simulink model "Torque_Vectoring_Schanzer20"  (R2018a)
settings: Solver=ode15s  StartTime=0.01  StopTime=inf  RelTol=1e-3  EnableMultiTasking=on
libraries: CarMaker4SL x8, dspstat3 x5, simulink x2
(part 2 of 3)

== system Torque_Vectoring_Schanzer20/CarMaker/IPG Vehicle/CarAndTrailer/Forces/Tires ==
  note: The TireXX_Out signals will only be used if FileIdent is "CarMaker-Tire-CM4SL" in the tire parameter file!
      | An example parameter file can be found in Data/Tire/DT_CM4SL_UserTire.
  Sync_In : Inport
  TireFL_In : Inport  Port=2
  TireFR_In : Inport  Port=3
  TireRL_In : Inport  Port=4
  TireRR_In : Inport  Port=5
  Bus Creator{1..4} (4 alike) : BusCreator  Inputs=11
  Demux{1..3,8} (4 alike) : Demux  Outputs=7
  TireFL : Subsystem
  TireFR : Subsystem
  TireRL : Subsystem
  TireRR : Subsystem
  TireFL_Out : Outport
  TireFR_Out : Outport  Port=2
  TireRL_Out : Outport  Port=3
  TireRR_Out : Outport  Port=4
  wires:
  Sync_In/1 -> TireRR/1(Sync_In), TireRL/1(Sync_In), TireFR/1(Sync_In), TireFL/1(Sync_In)
  Bus Creator4/1 -> TireRR_Out/1
  Bus Creator2/1 -> TireRL_Out/1
  Bus Creator1/1 -> TireFR_Out/1
  Demux3/5 -> TireRR/6(Rim_turnv)  "Tire_In Rim_turnv"
  Demux3/4 -> TireRR/5(Rim_rotv)  "Tire_In Rim_rotv"
  Demux3/1 -> TireRR/2(Load)  "Tire_In Load"
  Demux3/7 -> TireRR/8(muRoad)  "Tire_In mu"
  Demux3/6 -> TireRR/7(InclinAngle)  "Tire_In Camber"
  Demux3/2 -> TireRR/3(vxtrans)  "Tire_In vxtrans"
  Demux3/3 -> TireRR/4(vytrans)  "Tire_In vytrans"
  TireRR/11(AlignTrq) -> Bus Creator4/11  "Tire_Out AlignTrq"
  TireRR/10(RollResist) -> Bus Creator4/10  "Tire_Out RollResist"
  TireRR/9(OverturnTrq) -> Bus Creator4/9  "Tire_Out OverturnTrq"
  TireRR/8(LoadFrc) -> Bus Creator4/8  "Tire_Out LoadFrc"
  TireRR/7(SideFrc) -> Bus Creator4/7  "Tire_Out SideFrc"
  TireRR/6(LongFrc) -> Bus Creator4/6  "Tire_Out LongFrc"
  TireRR/5(vBelt) -> Bus Creator4/5  "Tire_Out vBelt"
  TireRR/4(rBelt_eff) -> Bus Creator4/4  "Tire_Out rBelt_eff"
  TireRR/3(TurnSlp) -> Bus Creator4/3  "Tire_Out TurnSlp"
  TireRR/1(Slp) -> Bus Creator4/1  "Tire_Out Slp"
  TireRR/2(Alpha) -> Bus Creator4/2  "Tire_Out Alpha"
  Demux2/5 -> TireRL/6(Rim_turnv)  "Tire_In Rim_turnv"
  Demux2/4 -> TireRL/5(Rim_rotv)  "Tire_In Rim_rotv"
  Demux2/1 -> TireRL/2(Load)  "Tire_In Load"
  Demux2/7 -> TireRL/8(muRoad)  "Tire_In mu"
  Demux2/6 -> TireRL/7(InclinAngle)  "Tire_In Camber"
  Demux2/2 -> TireRL/3(vxtrans)  "Tire_In vxtrans"
  Demux2/3 -> TireRL/4(vytrans)  "Tire_In vytrans"
  TireRL/11(AlignTrq) -> Bus Creator2/11  "Tire_Out AlignTrq"
  TireRL/10(RollResist) -> Bus Creator2/10  "Tire_Out RollResist"
  TireRL/9(OverturnTrq) -> Bus Creator2/9  "Tire_Out OverturnTrq"
  TireRL/8(LoadFrc) -> Bus Creator2/8  "Tire_Out LoadFrc"
  TireRL/7(SideFrc) -> Bus Creator2/7  "Tire_Out SideFrc"
  TireRL/6(LongFrc) -> Bus Creator2/6  "Tire_Out LongFrc"
  TireRL/5(vBelt) -> Bus Creator2/5  "Tire_Out vBelt"
  TireRL/4(rBelt_eff) -> Bus Creator2/4  "Tire_Out rBelt_eff"
  TireRL/3(TurnSlp) -> Bus Creator2/3  "Tire_Out TurnSlp"
  TireRL/1(Slp) -> Bus Creator2/1  "Tire_Out Slp"
  TireRL/2(Alpha) -> Bus Creator2/2  "Tire_Out Alpha"
  Demux1/5 -> TireFR/6(Rim_turnv)  "Tire_In Rim_turnv"
  Demux1/4 -> TireFR/5(Rim_rotv)  "Tire_In Rim_rotv"
  Demux1/1 -> TireFR/2(Load)  "Tire_In Load"
  Demux1/7 -> TireFR/8(muRoad)  "Tire_In mu"
  Demux1/6 -> TireFR/7(InclinAngle)  "Tire_In Camber"
  Demux1/2 -> TireFR/3(vxtrans)  "Tire_In vxtrans"
  Demux1/3 -> TireFR/4(vytrans)  "Tire_In vytrans"
  TireFR/11(AlignTrq) -> Bus Creator1/11  "Tire_Out AlignTrq"
  TireFR/10(RollResist) -> Bus Creator1/10  "Tire_Out RollResist"
  TireFR/9(OverturnTrq) -> Bus Creator1/9  "Tire_Out OverturnTrq"
  TireFR/8(LoadFrc) -> Bus Creator1/8  "Tire_Out LoadFrc"
  TireFR/7(SideFrc) -> Bus Creator1/7  "Tire_Out SideFrc"
  TireFR/6(LongFrc) -> Bus Creator1/6  "Tire_Out LongFrc"
  TireFR/5(vBelt) -> Bus Creator1/5  "Tire_Out vBelt"
  TireFR/4(rBelt_eff) -> Bus Creator1/4  "Tire_Out rBelt_eff"
  TireFR/3(TurnSlp) -> Bus Creator1/3  "Tire_Out TurnSlp"
  TireFR/1(Slp) -> Bus Creator1/1  "Tire_Out Slp"
  TireFR/2(Alpha) -> Bus Creator1/2  "Tire_Out Alpha"
  Demux8/5 -> TireFL/6(Rim_turnv)  "Tire_In Rim_turnv"
  Demux8/4 -> TireFL/5(Rim_rotv)  "Tire_In Rim_rotv"
  TireFL_In/1 -> Demux8/1
  Demux8/1 -> TireFL/2(Load)  "Tire_In Load"
  Demux8/7 -> TireFL/8(muRoad)  "Tire_In mu"
  Demux8/6 -> TireFL/7(InclinAngle)  "Tire_In Camber"
  Demux8/2 -> TireFL/3(vxtrans)  "Tire_In vxtrans"
  Demux8/3 -> TireFL/4(vytrans)  "Tire_In vytrans"
  TireFL/11(AlignTrq) -> Bus Creator3/11  "Tire_Out AlignTrq"
  TireFL/10(RollResist) -> Bus Creator3/10  "Tire_Out RollResist"
  TireFL/9(OverturnTrq) -> Bus Creator3/9  "Tire_Out OverturnTrq"
  TireFL/8(LoadFrc) -> Bus Creator3/8  "Tire_Out LoadFrc"
  TireFL/7(SideFrc) -> Bus Creator3/7  "Tire_Out SideFrc"
  TireFL/6(LongFrc) -> Bus Creator3/6  "Tire_Out LongFrc"
  TireFL/5(vBelt) -> Bus Creator3/5  "Tire_Out vBelt"
  TireFL/4(rBelt_eff) -> Bus Creator3/4  "Tire_Out rBelt_eff"
  TireFL/3(TurnSlp) -> Bus Creator3/3  "Tire_Out TurnSlp"
  TireFL/1(Slp) -> Bus Creator3/1  "Tire_Out Slp"
  TireFL/2(Alpha) -> Bus Creator3/2  "Tire_Out Alpha"
  Bus Creator3/1 -> TireFL_Out/1
  TireFR_In/1 -> Demux1/1
  TireRL_In/1 -> Demux2/1
  TireRR_In/1 -> Demux3/1

== system Torque_Vectoring_Schanzer20/CarMaker/IPG Vehicle/CarAndTrailer/Forces/Vehicle Forces ==
  Sync_In : Inport
  Bus Creator1 : BusCreator  Inputs=12
  Bus Creator8 : BusCreator  Inputs=16
  BusCreator1 : BusCreator  Inputs=4
  BusCreator2 : BusCreator  Inputs=9
  Demux : Demux  Outputs=16
  Demux1 : Demux  Outputs=12
  Demux2 : Demux  Outputs=13
  Forces : S-Function  FunctionName=CM_Sfun  Parameters='Forces'  SFunctionDeploymentMode=off  EnableBusSupport=off
  Terminator : Terminator
  Sync_Out : Outport
  Car.Virtual : Outport  Port=2
  Car.Aero : Outport  Port=3
  Car.Load : Outport  Port=4
  wires:
  BusCreator1/1 -> Terminator/1  "Aero IF (in)"
  Demux2/13 -> BusCreator2/9  "car Aero Trq_1 z"
  Demux2/12 -> BusCreator2/8  "car Aero Trq_1 y"
  Demux2/11 -> BusCreator2/7  "car Aero Trq_1 x"
  Demux2/10 -> BusCreator2/6  "car Aero Frc_1 z"
  Demux2/9 -> BusCreator2/5  "car Aero Frc_1 y"
  Demux2/8 -> BusCreator2/4  "car Aero Frc_1 x"
  Demux2/7 -> BusCreator2/3  "car Aero PoA_1 z"
  Demux2/6 -> BusCreator2/2  "car Aero PoA_1 y"
  Demux2/5 -> BusCreator2/1  "car Aero PoA_1 x"
  Demux2/4 -> BusCreator1/4  "car Aero tau_1"
  Demux2/3 -> BusCreator1/3  "car Aero ApproachVel_1 z"
  Demux2/2 -> BusCreator1/2  "car Aero ApproachVel_1 y"
  Demux2/1 -> BusCreator1/1  "car Aero ApproachVel_1 x"
  Demux/16 -> Bus Creator8/16  "Car Load_3 tz"
  Demux/15 -> Bus Creator8/15  "Car Load_3 ty"
  Demux/14 -> Bus Creator8/14  "Car Load_3 tx"
  Demux/13 -> Bus Creator8/13  "Car Load_3 mass"
  Demux1/12 -> Bus Creator1/12  "Car Virtual Trq_0 z"
  Demux1/11 -> Bus Creator1/11  "Car Virtual Trq_0 y"
  Demux1/10 -> Bus Creator1/10  "Car Virtual Trq_0 x"
  Demux1/9 -> Bus Creator1/9  "Car Virtual Trq_1 z"
  Demux1/8 -> Bus Creator1/8  "Car Virtual Trq_1 y"
  Demux1/7 -> Bus Creator1/7  "Car Virtual Trq_1 x"
  Demux1/6 -> Bus Creator1/6  "Car Virtual Frc_0 z"
  Demux1/5 -> Bus Creator1/5  "Car Virtual Frc_0 y"
  Demux1/4 -> Bus Creator1/4  "Car Virtual Frc_0 x"
  Sync_In/1 -> Forces/1
  Forces/1 -> Sync_Out/1
  BusCreator2/1 -> Car.Aero/1
  Demux1/1 -> Bus Creator1/1  "Car Virtual Frc_1 x"
  Demux1/2 -> Bus Creator1/2  "Car Virtual Frc_1 y"
  Demux1/3 -> Bus Creator1/3  "Car Virtual Frc_1 z"
  Forces/3 -> Demux2/1
  Forces/2 -> Demux1/1
  Bus Creator1/1 -> Car.Virtual/1
  Bus Creator8/1 -> Car.Load/1
  Demux/1 -> Bus Creator8/1  "Car Load_0 mass"
  Demux/2 -> Bus Creator8/2  "Car Load_0 tx"
  Demux/3 -> Bus Creator8/3  "Car Load_0 ty"
  Demux/4 -> Bus Creator8/4  "Car Load_0 tz"
  Demux/5 -> Bus Creator8/5  "Car Load_1 mass"
  Demux/6 -> Bus Creator8/6  "Car Load_1 tx"
  Demux/7 -> Bus Creator8/7  "Car Load_1 ty"
  Demux/8 -> Bus Creator8/8  "Car Load_1 tz"
  Demux/9 -> Bus Creator8/9  "Car Load_2 mass"
  Demux/10 -> Bus Creator8/10  "Car Load_2 tx"
  Demux/11 -> Bus Creator8/11  "Car Load_2 ty"
  Demux/12 -> Bus Creator8/12  "Car Load_2 tz"
  Forces/4 -> Demux/1

== system Torque_Vectoring_Schanzer20/CarMaker/IPG Vehicle/CarAndTrailer/Trailer/CreateBus Car.Hitch.FrcTrq ==
  In1 : Inport
  Bus Creator7 : BusCreator  Inputs=6
  Demux7 : Demux  Outputs=6
  Out1 : Outport
  wires:
  In1/1 -> Demux7/1
  Bus Creator7/1 -> Out1/1
  Demux7/6 -> Bus Creator7/6  "Car Hitch Trq2Car z"
  Demux7/5 -> Bus Creator7/5  "Car Hitch Trq2Car y"
  Demux7/4 -> Bus Creator7/4  "Car Hitch Trq2Car x"
  Demux7/3 -> Bus Creator7/3  "Car Hitch Frc2Car z"
  Demux7/2 -> Bus Creator7/2  "Car Hitch Frc2Car y"
  Demux7/1 -> Bus Creator7/1  "Car Hitch Frc2Car x"

== system Torque_Vectoring_Schanzer20/CarMaker/IPG Vehicle/CarAndTrailer/Trailer/CreateBus Vhcl.Motion ==
  In1 : Inport
  BusCreator : BusCreator  Inputs=15
  Demux : Demux  Outputs=15
  Scope : Scope
  Out1 : Outport
  Out2 : Outport  Port=2
  Out3 : Outport  Port=3
  wires:
  Demux/15 -> BusCreator/15  "Vhcl YawAcc"
  Demux/14 -> Scope/1, Out3/1, BusCreator/14  "Vhcl YawVel"
  Demux/13 -> BusCreator/13  "Vhcl Yaw"
  Demux/12 -> BusCreator/12  "Vhcl PitchAcc"
  Demux/11 -> BusCreator/11  "Vhcl PitchVel"
  Demux/10 -> BusCreator/10  "Vhcl Pitch"
  Demux/9 -> BusCreator/9  "Vhcl RollAcc"
  Demux/8 -> BusCreator/8  "Vhcl RollVel"
  Demux/7 -> BusCreator/7  "Vhcl Roll"
  Demux/6 -> BusCreator/6  "Vhcl Hitch_Pos z"
  Demux/5 -> BusCreator/5  "Vhcl Hitch_Pos y"
  Demux/4 -> BusCreator/4  "Vhcl Hitch_Pos x"
  Demux/3 -> BusCreator/3  "Vhcl sRoad"
  Demux/2 -> BusCreator/2  "Vhcl Distance"
  Demux/1 -> Out2/1, BusCreator/1  "Vhcl v"
  In1/1 -> Demux/1
  BusCreator/1 -> Out1/1

== system Torque_Vectoring_Schanzer20/CarMaker/IPG Vehicle/CarAndTrailer/Trailer/CreateBus Vhcl.PoI ==
  In1 : Inport
  Bus Creator3 : BusCreator  Inputs=18
  Demux3 : Demux  Outputs=18
  Out1 : Outport
  Out2 : Outport  Port=2
  wires:
  Demux3/18 -> Bus Creator3/18  "Vhcl PoI_GCS Elev"
  Demux3/17 -> Bus Creator3/17  "Vhcl PoI_GCS Lat"
  Demux3/16 -> Bus Creator3/16  "Vhcl PoI_GCS Long"
  Demux3/15 -> Bus Creator3/15  "Vhcl PoI_Acc_1 z"
  Demux3/14 -> Bus Creator3/14  "Vhcl PoI_Acc_1 y"
  Demux3/13 -> Out2/1, Bus Creator3/13  "Vhcl PoI_Acc_1 x"
  Demux3/12 -> Bus Creator3/12  "Vhcl PoI_Vel_1 z"
  Demux3/11 -> Bus Creator3/11  "Vhcl PoI_Vel_1 y"
  Demux3/10 -> Bus Creator3/10  "Vhcl PoI_Vel_1 x"
  Demux3/9 -> Bus Creator3/9  "Vhcl PoI_Acc z"
  Demux3/8 -> Bus Creator3/8  "Vhcl PoI_Acc y"
  Demux3/7 -> Bus Creator3/7  "Vhcl PoI_Acc x"
  Demux3/6 -> Bus Creator3/6  "Vhcl PoI_Vel z"
  Demux3/5 -> Bus Creator3/5  "Vhcl PoI_Vel y"
  Demux3/4 -> Bus Creator3/4  "Vhcl PoI_Vel x"
  Demux3/3 -> Bus Creator3/3  "Vhcl PoI_Pos z"
  Demux3/2 -> Bus Creator3/2  "Vhcl PoI_Pos y"
  In1/1 -> Demux3/1
  Bus Creator3/1 -> Out1/1
  Demux3/1 -> Bus Creator3/1  "Vhcl PoI_Pos x"

== system Torque_Vectoring_Schanzer20/CarMaker/IPG Vehicle/CarAndTrailer/Trailer/CreateBus Vhcl.Steering ==
  In1 : Inport
  Bus Creator3 : BusCreator  Inputs=4
  Demux : Demux
  Out1 : Outport
  Out2 : Outport  Port=2
  wires:
  Bus Creator3/1 -> Out1/1
  Demux/1 -> Out2/1, Bus Creator3/1  "Vehicle Steering Ang"
  Demux/3 -> Bus Creator3/3  "Vhcl Steering AngAcc"
  Demux/2 -> Bus Creator3/2  "Vhcl Steering AngVel"
  Demux/4 -> Bus Creator3/4  "Vhcl Steering Trq"
  In1/1 -> Demux/1

== system Torque_Vectoring_Schanzer20/CarMaker/IPG Vehicle/CarAndTrailer/Trailer/CreateBus Vhcl.Wheel.FL ==
  In1 : Inport
  Bus Creator3 : BusCreator  Inputs=14
  Demux3 : Demux  Outputs=14
  Out1 : Outport
  wires:
  Demux3/14 -> Bus Creator3/14  "Vhcl Wheel FL Trq_WhlBearing"
  Demux3/12 -> Bus Creator3/12  "Vhcl Wheel FL SideSlip"
  Demux3/11 -> Bus Creator3/11  "Vhcl Wheel FL LongSlip"
  Demux3/10 -> Bus Creator3/10  "Vhcl Wheel FL vBelt"
  Demux3/9 -> Bus Creator3/9  "Vhcl Wheel FL Fz"
  Demux3/8 -> Bus Creator3/8  "Vhcl Wheel FL Fy"
  Demux3/7 -> Bus Creator3/7  "Vhcl Wheel FL Fx"
  Demux3/6 -> Bus Creator3/6  "Vhcl Wheel FL r_zxy z"
  Demux3/5 -> Bus Creator3/5  "Vhcl Wheel FL r_zxy y"
  Demux3/4 -> Bus Creator3/4  "Vhcl Wheel FL r_zxy x"
  Demux3/3 -> Bus Creator3/3  "Vhcl Wheel FL t z"
  Demux3/2 -> Bus Creator3/2  "Vhcl Wheel FL t y"
  In1/1 -> Demux3/1
  Bus Creator3/1 -> Out1/1
  Demux3/1 -> Bus Creator3/1  "Vhcl Wheel FL t x"
  Demux3/13 -> Bus Creator3/13  "Vhcl Wheel FL Trq_T2W"

== system Torque_Vectoring_Schanzer20/CarMaker/IPG Vehicle/CarAndTrailer/Trailer/CreateBus Vhcl.Wheel.FR ==
  In1 : Inport
  Bus Creator3 : BusCreator  Inputs=14
  Demux3 : Demux  Outputs=14
  Out1 : Outport
  wires:
  Demux3/14 -> Bus Creator3/14  "Vhcl Wheel FR Trq_WhlBearing"
  Demux3/12 -> Bus Creator3/12  "Vhcl Wheel FR SideSlip"
  Demux3/11 -> Bus Creator3/11  "Vhcl Wheel FR LongSlip"
  Demux3/10 -> Bus Creator3/10  "Vhcl Wheel FR vBelt"
  Demux3/9 -> Bus Creator3/9  "Vhcl Wheel FR Fz"
  Demux3/8 -> Bus Creator3/8  "Vhcl Wheel FR Fy"
  Demux3/7 -> Bus Creator3/7  "Vhcl Wheel FR Fx"
  Demux3/6 -> Bus Creator3/6  "Vhcl Wheel FR r_zxy z"
  Demux3/5 -> Bus Creator3/5  "Vhcl Wheel FR r_zxy y"
  Demux3/4 -> Bus Creator3/4  "Vhcl Wheel FR r_zxy x"
  Demux3/3 -> Bus Creator3/3  "Vhcl Wheel FR t z"
  Demux3/2 -> Bus Creator3/2  "Vhcl Wheel FR t y"
  In1/1 -> Demux3/1
  Bus Creator3/1 -> Out1/1
  Demux3/1 -> Bus Creator3/1  "Vhcl Wheel FR t x"
  Demux3/13 -> Bus Creator3/13  "Vhcl Wheel FR Trq_T2W"

== system Torque_Vectoring_Schanzer20/CarMaker/IPG Vehicle/CarAndTrailer/Trailer/CreateBus Vhcl.Wheel.RL ==
  In1 : Inport
  Bus Creator3 : BusCreator  Inputs=14
  Demux3 : Demux  Outputs=14
  Out1 : Outport
  wires:
  Demux3/14 -> Bus Creator3/14  "Vhcl Wheel RL Trq_WhlBearing"
  Demux3/12 -> Bus Creator3/12  "Vhcl Wheel RL SideSlip"
  Demux3/11 -> Bus Creator3/11  "Vhcl Wheel RL LongSlip"
  Demux3/10 -> Bus Creator3/10  "Vhcl Wheel RL vBelt"
  Demux3/9 -> Bus Creator3/9  "Vhcl Wheel RL Fz"
  Demux3/8 -> Bus Creator3/8  "Vhcl Wheel RL Fy"
  Demux3/7 -> Bus Creator3/7  "Vhcl Wheel RL Fx"
  Demux3/6 -> Bus Creator3/6  "Vhcl Wheel RL r_zxy z"
  Demux3/5 -> Bus Creator3/5  "Vhcl Wheel RL r_zxy y"
  Demux3/4 -> Bus Creator3/4  "Vhcl Wheel RL r_zxy x"
  Demux3/3 -> Bus Creator3/3  "Vhcl Wheel RL t z"
  Demux3/2 -> Bus Creator3/2  "Vhcl Wheel RL t y"
  In1/1 -> Demux3/1
  Bus Creator3/1 -> Out1/1
  Demux3/1 -> Bus Creator3/1  "Vhcl Wheel RL t x"
  Demux3/13 -> Bus Creator3/13  "Vhcl Wheel RL Trq_T2W"

== system Torque_Vectoring_Schanzer20/CarMaker/IPG Vehicle/CarAndTrailer/Trailer/CreateBus Vhcl.Wheel.RR ==
  In1 : Inport
  Bus Creator3 : BusCreator  Inputs=14
  Demux3 : Demux  Outputs=14
  Out1 : Outport
  wires:
  Demux3/14 -> Bus Creator3/14  "Vhcl Wheel RR Trq_WhlBearing"
  Demux3/12 -> Bus Creator3/12  "Vhcl Wheel RR SideSlip"
  Demux3/11 -> Bus Creator3/11  "Vhcl Wheel RR LongSlip"
  Demux3/10 -> Bus Creator3/10  "Vhcl Wheel RR vBelt"
  Demux3/9 -> Bus Creator3/9  "Vhcl Wheel RR Fz"
  Demux3/8 -> Bus Creator3/8  "Vhcl Wheel RR Fy"
  Demux3/7 -> Bus Creator3/7  "Vhcl Wheel RR Fx"
  Demux3/6 -> Bus Creator3/6  "Vhcl Wheel RR r_zxy z"
  Demux3/5 -> Bus Creator3/5  "Vhcl Wheel RR r_zxy y"
  Demux3/4 -> Bus Creator3/4  "Vhcl Wheel RR r_zxy x"
  Demux3/3 -> Bus Creator3/3  "Vhcl Wheel RR t z"
  Demux3/2 -> Bus Creator3/2  "Vhcl Wheel RR t y"
  In1/1 -> Demux3/1
  Bus Creator3/1 -> Out1/1
  Demux3/1 -> Bus Creator3/1  "Vhcl Wheel RR t x"
  Demux3/13 -> Bus Creator3/13  "Vhcl Wheel RR Trq_T2W"

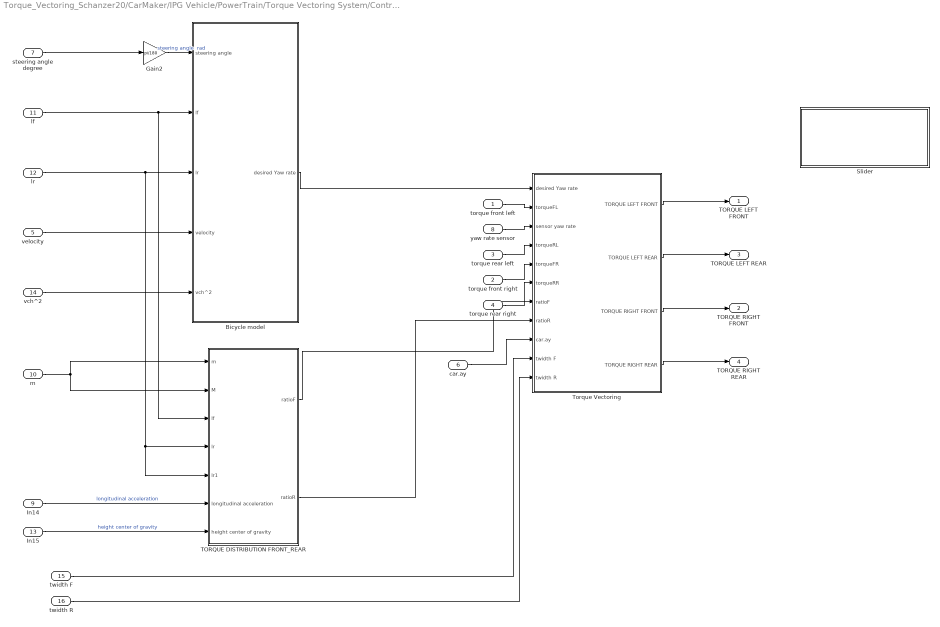
== system Torque_Vectoring_Schanzer20/CarMaker/IPG Vehicle/PowerTrain/Torque Vectoring System/Controller Logic1 ==
  torque front left : Inport
  torque front right : Inport  Port=2
  torque rear left : Inport  Port=3
  torque rear right : Inport  Port=4
  velocity : Inport  Port=5
  car.ay : Inport  Port=6
  steering angle degree : Inport  Port=7
  yaw rate sensor : Inport  Port=8
  In14 : Inport  Port=9
  m : Inport  Port=10
  lf : Inport  Port=11
  lr : Inport  Port=12
  In15 : Inport  Port=13
  vch^2 : Inport  Port=14
  twidth F : Inport  Port=15
  twidth R : Inport  Port=16
  Bicycle model : Subsystem
  Gain2 : Gain  Gain=pi/180
  Slider : Subsystem  DialogController=hmiCreateDDGDialog  IsWebBlock=on  mask(MWDashboardBlock){webBlockId=59816ab4-1199-4927-a44c-d672ac8afe40, webBlockType=slider, ShowInLibBrowser=on, ShowInitialText=on, HMISrcModelName=Torque_Vectoring_Schanzer20}
      mask prompts: webBlockId "WebBlock Id"; webBlockType "WebBlock Type"; HMISrcModelName "Source Model"
      mask help: SimulinkHMI:dialogs:SliderDialogDesc
      mask Help: helpview([docroot '/mapfiles/simulink.map'], 'hmi_slider')
      mask Display:
      | if strcmp(get_param(bdroot(gcb),'BlockDiagramType'), 'library')
      |     image([(matlabroot) '/toolbox/simulink/hmi/icons/Slider.png']);
      | end
  TORQUE DISTRIBUTION FRONT_REAR : Subsystem
  Torque Vectoring : Subsystem
  TORQUE LEFT FRONT : Outport
  TORQUE RIGHT FRONT : Outport  Port=2
  TORQUE LEFT REAR : Outport  Port=3
  TORQUE RIGHT REAR : Outport  Port=4
  wires:
  Gain2/1 -> Bicycle model/1(steering angle)  "steering angle  rad"
  steering angle degree/1 -> Gain2/1
  lf/1 -> TORQUE DISTRIBUTION FRONT_REAR/3(lf), Bicycle model/2(lf)
  m/1 -> TORQUE DISTRIBUTION FRONT_REAR/2(M), TORQUE DISTRIBUTION FRONT_REAR/1(m)
  lr/1 -> TORQUE DISTRIBUTION FRONT_REAR/5(lr1), TORQUE DISTRIBUTION FRONT_REAR/4(lr), Bicycle model/3(lr)
  In14/1 -> TORQUE DISTRIBUTION FRONT_REAR/6(longitudinal acceleration)  "longitudinal acceleration"
  In15/1 -> TORQUE DISTRIBUTION FRONT_REAR/7(height center of gravity)  "height center of gravity"
  velocity/1 -> Bicycle model/4(velocity)
  Bicycle model/1(" desired Yaw rate") -> Torque Vectoring/1(desired Yaw rate)
  torque front left/1 -> Torque Vectoring/2(torqueFL)
  yaw rate sensor/1 -> Torque Vectoring/3(sensor yaw rate)
  torque rear left/1 -> Torque Vectoring/4(torqueRL)
  torque front right/1 -> Torque Vectoring/5(torqueFR)
  torque rear right/1 -> Torque Vectoring/6(torqueRR)
  TORQUE DISTRIBUTION FRONT_REAR/1(ratioF) -> Torque Vectoring/7(ratioF)
  TORQUE DISTRIBUTION FRONT_REAR/2(ratioR) -> Torque Vectoring/8(ratioR)
  Torque Vectoring/1(TORQUE LEFT FRONT) -> TORQUE LEFT FRONT/1
  Torque Vectoring/2(TORQUE LEFT REAR) -> TORQUE LEFT REAR/1
  Torque Vectoring/3(TORQUE RIGHT FRONT) -> TORQUE RIGHT FRONT/1
  Torque Vectoring/4(TORQUE RIGHT REAR) -> TORQUE RIGHT REAR/1
  car.ay/1 -> Torque Vectoring/9(car.ay)
  vch^2/1 -> Bicycle model/5(vch^2)
  twidth F/1 -> Torque Vectoring/10(twidth F)
  twidth R/1 -> Torque Vectoring/11(twidth R)

== system Torque_Vectoring_Schanzer20/CarMaker/IPG Vehicle/PowerTrain/Torque Vectoring System/activate system dependent1 ==
  In1 : Inport
  Constant1 : Constant  Value=0
  If : If  IfExpression=u1 > 0.1
  If Action Subsystem : Subsystem  TreatAsAtomicUnit=on
  If Action Subsystem1 : Subsystem  TreatAsAtomicUnit=on
  If Action Subsystem2 : Subsystem  TreatAsAtomicUnit=on
  If Action Subsystem3 : Subsystem  TreatAsAtomicUnit=on
  If1 : If  IfExpression=u1 < 1000
  Merge : Merge  InitialOutput=0
  Merge1 : Merge  InitialOutput=0
  Out1 : Outport
  wires:
  If Action Subsystem3/1(Out1) -> Merge1/2
  If/1 -> If Action Subsystem/Action
  Constant1/1 -> If Action Subsystem3/1(In1), If Action Subsystem1/1(In1)
  If Action Subsystem/1(Out1) -> Merge/1
  In1/1 -> If Action Subsystem/1(In1), If/1, If1/1
  If1/1 -> If Action Subsystem2/Action
  If Action Subsystem1/1(Out1) -> Merge/2
  If1/2 -> If Action Subsystem3/Action
  If/2 -> If Action Subsystem1/Action
  If Action Subsystem2/1(Out1) -> Merge1/1
  Merge/1 -> If Action Subsystem2/1(In1)
  Merge1/1 -> Out1/1

== system Torque_Vectoring_Schanzer20/CarMaker/IPG Vehicle/PowerTrain/Torque Vectoring System/activate system dependent2 ==
  In1 : Inport
  Constant1 : Constant  Value=0
  If : If  IfExpression=u1 > 0.1
  If Action Subsystem : Subsystem  TreatAsAtomicUnit=on
  If Action Subsystem1 : Subsystem  TreatAsAtomicUnit=on
  If Action Subsystem2 : Subsystem  TreatAsAtomicUnit=on
  If Action Subsystem3 : Subsystem  TreatAsAtomicUnit=on
  If1 : If  IfExpression=u1 < 1000
  Merge : Merge  InitialOutput=0
  Merge1 : Merge  InitialOutput=0
  Out1 : Outport
  wires:
  If Action Subsystem3/1(Out1) -> Merge1/2
  If/1 -> If Action Subsystem/Action
  Constant1/1 -> If Action Subsystem3/1(In1), If Action Subsystem1/1(In1)
  If Action Subsystem/1(Out1) -> Merge/1
  In1/1 -> If Action Subsystem/1(In1), If/1, If1/1
  If1/1 -> If Action Subsystem2/Action
  If Action Subsystem1/1(Out1) -> Merge/2
  If1/2 -> If Action Subsystem3/Action
  If/2 -> If Action Subsystem1/Action
  If Action Subsystem2/1(Out1) -> Merge1/1
  Merge/1 -> If Action Subsystem2/1(In1)
  Merge1/1 -> Out1/1

== system Torque_Vectoring_Schanzer20/CarMaker/IPG Vehicle/PowerTrain/Torque Vectoring System/activate system dependent3 ==
  In1 : Inport
  Constant1 : Constant  Value=0
  If : If  IfExpression=u1 > 0.1
  If Action Subsystem : Subsystem  TreatAsAtomicUnit=on
  If Action Subsystem1 : Subsystem  TreatAsAtomicUnit=on
  If Action Subsystem2 : Subsystem  TreatAsAtomicUnit=on
  If Action Subsystem3 : Subsystem  TreatAsAtomicUnit=on
  If1 : If  IfExpression=u1 < 1000
  Merge : Merge  InitialOutput=0
  Merge1 : Merge  InitialOutput=0
  Out1 : Outport
  wires:
  If Action Subsystem3/1(Out1) -> Merge1/2
  If/1 -> If Action Subsystem/Action
  Constant1/1 -> If Action Subsystem3/1(In1), If Action Subsystem1/1(In1)
  If Action Subsystem/1(Out1) -> Merge/1
  In1/1 -> If Action Subsystem/1(In1), If/1, If1/1
  If1/1 -> If Action Subsystem2/Action
  If Action Subsystem1/1(Out1) -> Merge/2
  If1/2 -> If Action Subsystem3/Action
  If/2 -> If Action Subsystem1/Action
  If Action Subsystem2/1(Out1) -> Merge1/1
  Merge/1 -> If Action Subsystem2/1(In1)
  Merge1/1 -> Out1/1

== system Torque_Vectoring_Schanzer20/CarMaker/IPG Vehicle/PowerTrain/Torque Vectoring System/activate system dependent5 ==
  In1 : Inport
  Constant1 : Constant
  If : If  IfExpression=u1 > 0.01
  If Action Subsystem : Subsystem  TreatAsAtomicUnit=on
  If Action Subsystem1 : Subsystem  TreatAsAtomicUnit=on
  If Action Subsystem2 : Subsystem  TreatAsAtomicUnit=on
  If Action Subsystem3 : Subsystem  TreatAsAtomicUnit=on
  If1 : If  IfExpression=u1 < 1000
  Merge : Merge  InitialOutput=0
  Merge1 : Merge  InitialOutput=0
  Out1 : Outport
  wires:
  If Action Subsystem3/1(Out1) -> Merge1/2
  If/1 -> If Action Subsystem/Action
  Constant1/1 -> If Action Subsystem3/1(In1), If Action Subsystem1/1(In1)
  If Action Subsystem/1(Out1) -> Merge/1
  In1/1 -> If Action Subsystem/1(In1), If/1, If1/1
  If1/1 -> If Action Subsystem2/Action
  If Action Subsystem1/1(Out1) -> Merge/2
  If1/2 -> If Action Subsystem3/Action
  If/2 -> If Action Subsystem1/Action
  If Action Subsystem2/1(Out1) -> Merge1/1
  Merge/1 -> If Action Subsystem2/1(In1)
  Merge1/1 -> Out1/1

== system Torque_Vectoring_Schanzer20/CarMaker/IPG Vehicle/PowerTrain/Torque Vectoring System/activate system dependent6 ==
  In1 : Inport
  Constant1 : Constant  Value=0
  If : If  IfExpression=u1 > 0.1
  If Action Subsystem : Subsystem  TreatAsAtomicUnit=on
  If Action Subsystem1 : Subsystem  TreatAsAtomicUnit=on
  If Action Subsystem2 : Subsystem  TreatAsAtomicUnit=on
  If Action Subsystem3 : Subsystem  TreatAsAtomicUnit=on
  If1 : If  IfExpression=u1 < 1000
  Merge : Merge  InitialOutput=0
  Merge1 : Merge  InitialOutput=0
  Out1 : Outport
  wires:
  If Action Subsystem3/1(Out1) -> Merge1/2
  If/1 -> If Action Subsystem/Action
  Constant1/1 -> If Action Subsystem3/1(In1), If Action Subsystem1/1(In1)
  If Action Subsystem/1(Out1) -> Merge/1
  In1/1 -> If Action Subsystem/1(In1), If/1, If1/1
  If1/1 -> If Action Subsystem2/Action
  If Action Subsystem1/1(Out1) -> Merge/2
  If1/2 -> If Action Subsystem3/Action
  If/2 -> If Action Subsystem1/Action
  If Action Subsystem2/1(Out1) -> Merge1/1
  Merge/1 -> If Action Subsystem2/1(In1)
  Merge1/1 -> Out1/1

== system Torque_Vectoring_Schanzer20/CarMaker/IPG Vehicle/PowerTrain/Torque Vectoring System/velocity estimation ==
  note: Assuming that angle of attack change rate is 0 -> steady state cornering (improvement would be including estimation of angle of attack (and change rate)
      | Checking of straight line noise of yaw rate sensor necessary to define a reasonable treshhold
  note: Ignore sensor offset; only switching when threshold is exceeded
  yaw rate : Inport
  centrifugal acceleration : Inport  Port=2
  Abs : Abs
  Abs1 : Abs
  Add : Sum
  Constant : Constant  Value=-1
  Constant1 : Constant  Value=-1
  Memory : Memory
  Sampling continous signal 50Hz1 : RateTransition  OutPortSampleTime=1/50
  Sampling continous signal 50Hz4 : RateTransition  OutPortSampleTime=1/50
  Switch1 : Switch  Criteria=u2 > Threshold  Threshold=0.05
  Switch2 : Switch  Criteria=u2 > Threshold  Threshold=0.1
  Switch3 : Switch
  v_viaYawRate_CentrifugalAcceleration : Subsystem
  Out1 : Outport
  wires:
  Add/1 -> Switch3/2
  Sampling continous signal 50Hz1/1 -> Switch1/2, Switch1/1
  Switch3/1 -> Out1/1, Memory/1  "velocity"
  Abs1/1 -> Sampling continous signal 50Hz4/1
  Switch1/1 -> Add/1, v_viaYawRate_CentrifugalAcceleration/1(YawRate)
  Sampling continous signal 50Hz4/1 -> Switch2/2, Switch2/1
  Memory/1 -> Switch3/3
  Abs/1 -> Sampling continous signal 50Hz1/1
  Constant1/1 -> Switch1/3
  yaw rate/1 -> Abs/1  "YawRate"
  v_viaYawRate_CentrifugalAcceleration/1(Out1) -> Switch3/1
  Constant/1 -> Switch2/3
  Switch2/1 -> Add/2, v_viaYawRate_CentrifugalAcceleration/2(ay)
  centrifugal acceleration/1 -> Abs1/1  "ay"

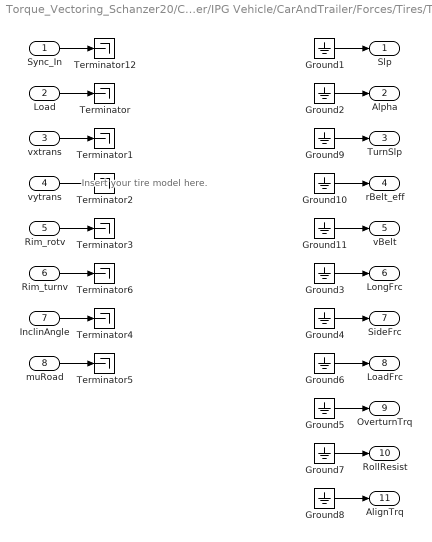
== system Torque_Vectoring_Schanzer20/CarMaker/IPG Vehicle/CarAndTrailer/Forces/Tires/TireFL ==
  note: Insert your tire model here.
  Sync_In : Inport
  Load : Inport  Port=2
  vxtrans : Inport  Port=3
  vytrans : Inport  Port=4
  Rim_rotv : Inport  Port=5
  Rim_turnv : Inport  Port=6
  InclinAngle : Inport  Port=7
  muRoad : Inport  Port=8
  Ground{1..11} (11 alike) : Ground
  Terminator{,1..6,12} (8 alike) : Terminator
  Slp : Outport
  Alpha : Outport  Port=2
  TurnSlp : Outport  Port=3
  rBelt_eff : Outport  Port=4
  vBelt : Outport  Port=5
  LongFrc : Outport  Port=6
  SideFrc : Outport  Port=7
  LoadFrc : Outport  Port=8
  OverturnTrq : Outport  Port=9
  RollResist : Outport  Port=10
  AlignTrq : Outport  Port=11
  wires:
  Ground11/1 -> vBelt/1
  Ground10/1 -> rBelt_eff/1
  Ground9/1 -> TurnSlp/1
  Rim_turnv/1 -> Terminator6/1
  Sync_In/1 -> Terminator12/1
  Ground2/1 -> Alpha/1
  Ground3/1 -> LongFrc/1
  Ground4/1 -> SideFrc/1
  Ground5/1 -> OverturnTrq/1
  vxtrans/1 -> Terminator1/1
  vytrans/1 -> Terminator2/1
  Rim_rotv/1 -> Terminator3/1
  InclinAngle/1 -> Terminator4/1
  muRoad/1 -> Terminator5/1
  Load/1 -> Terminator/1
  Ground1/1 -> Slp/1
  Ground6/1 -> LoadFrc/1
  Ground7/1 -> RollResist/1
  Ground8/1 -> AlignTrq/1

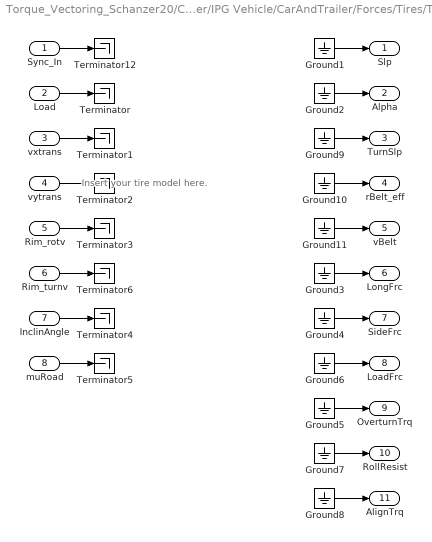
== system Torque_Vectoring_Schanzer20/CarMaker/IPG Vehicle/CarAndTrailer/Forces/Tires/TireFR ==
  note: Insert your tire model here.
  Sync_In : Inport
  Load : Inport  Port=2
  vxtrans : Inport  Port=3
  vytrans : Inport  Port=4
  Rim_rotv : Inport  Port=5
  Rim_turnv : Inport  Port=6
  InclinAngle : Inport  Port=7
  muRoad : Inport  Port=8
  Ground{1..11} (11 alike) : Ground
  Terminator{,1..6,12} (8 alike) : Terminator
  Slp : Outport
  Alpha : Outport  Port=2
  TurnSlp : Outport  Port=3
  rBelt_eff : Outport  Port=4
  vBelt : Outport  Port=5
  LongFrc : Outport  Port=6
  SideFrc : Outport  Port=7
  LoadFrc : Outport  Port=8
  OverturnTrq : Outport  Port=9
  RollResist : Outport  Port=10
  AlignTrq : Outport  Port=11
  wires:
  Ground11/1 -> vBelt/1
  Ground10/1 -> rBelt_eff/1
  Ground9/1 -> TurnSlp/1
  Rim_turnv/1 -> Terminator6/1
  Sync_In/1 -> Terminator12/1
  Ground2/1 -> Alpha/1
  Ground3/1 -> LongFrc/1
  Ground4/1 -> SideFrc/1
  Ground5/1 -> OverturnTrq/1
  vxtrans/1 -> Terminator1/1
  vytrans/1 -> Terminator2/1
  Rim_rotv/1 -> Terminator3/1
  InclinAngle/1 -> Terminator4/1
  muRoad/1 -> Terminator5/1
  Load/1 -> Terminator/1
  Ground1/1 -> Slp/1
  Ground6/1 -> LoadFrc/1
  Ground7/1 -> RollResist/1
  Ground8/1 -> AlignTrq/1

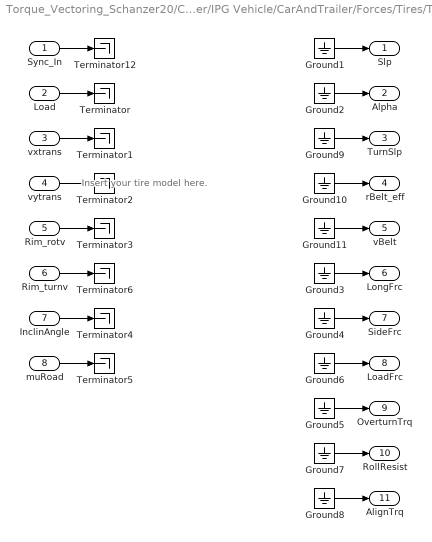
== system Torque_Vectoring_Schanzer20/CarMaker/IPG Vehicle/CarAndTrailer/Forces/Tires/TireRL ==
  note: Insert your tire model here.
  Sync_In : Inport
  Load : Inport  Port=2
  vxtrans : Inport  Port=3
  vytrans : Inport  Port=4
  Rim_rotv : Inport  Port=5
  Rim_turnv : Inport  Port=6
  InclinAngle : Inport  Port=7
  muRoad : Inport  Port=8
  Ground{1..11} (11 alike) : Ground
  Terminator{,1..6,12} (8 alike) : Terminator
  Slp : Outport
  Alpha : Outport  Port=2
  TurnSlp : Outport  Port=3
  rBelt_eff : Outport  Port=4
  vBelt : Outport  Port=5
  LongFrc : Outport  Port=6
  SideFrc : Outport  Port=7
  LoadFrc : Outport  Port=8
  OverturnTrq : Outport  Port=9
  RollResist : Outport  Port=10
  AlignTrq : Outport  Port=11
  wires:
  Ground11/1 -> vBelt/1
  Ground10/1 -> rBelt_eff/1
  Ground9/1 -> TurnSlp/1
  Rim_turnv/1 -> Terminator6/1
  Sync_In/1 -> Terminator12/1
  Ground2/1 -> Alpha/1
  Ground3/1 -> LongFrc/1
  Ground4/1 -> SideFrc/1
  Ground5/1 -> OverturnTrq/1
  vxtrans/1 -> Terminator1/1
  vytrans/1 -> Terminator2/1
  Rim_rotv/1 -> Terminator3/1
  InclinAngle/1 -> Terminator4/1
  muRoad/1 -> Terminator5/1
  Load/1 -> Terminator/1
  Ground1/1 -> Slp/1
  Ground6/1 -> LoadFrc/1
  Ground7/1 -> RollResist/1
  Ground8/1 -> AlignTrq/1

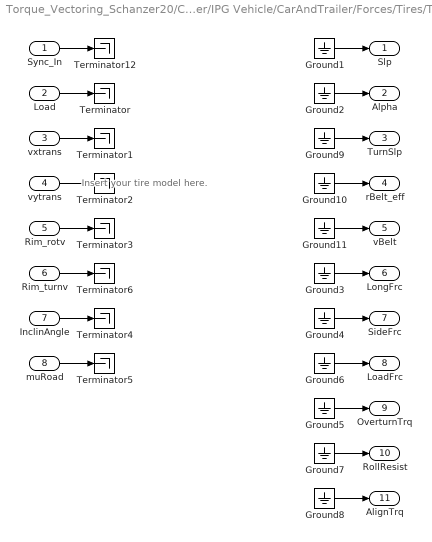
== system Torque_Vectoring_Schanzer20/CarMaker/IPG Vehicle/CarAndTrailer/Forces/Tires/TireRR ==
  note: Insert your tire model here.
  Sync_In : Inport
  Load : Inport  Port=2
  vxtrans : Inport  Port=3
  vytrans : Inport  Port=4
  Rim_rotv : Inport  Port=5
  Rim_turnv : Inport  Port=6
  InclinAngle : Inport  Port=7
  muRoad : Inport  Port=8
  Ground{1..11} (11 alike) : Ground
  Terminator{,1..6,12} (8 alike) : Terminator
  Slp : Outport
  Alpha : Outport  Port=2
  TurnSlp : Outport  Port=3
  rBelt_eff : Outport  Port=4
  vBelt : Outport  Port=5
  LongFrc : Outport  Port=6
  SideFrc : Outport  Port=7
  LoadFrc : Outport  Port=8
  OverturnTrq : Outport  Port=9
  RollResist : Outport  Port=10
  AlignTrq : Outport  Port=11
  wires:
  Ground11/1 -> vBelt/1
  Ground10/1 -> rBelt_eff/1
  Ground9/1 -> TurnSlp/1
  Rim_turnv/1 -> Terminator6/1
  Sync_In/1 -> Terminator12/1
  Ground2/1 -> Alpha/1
  Ground3/1 -> LongFrc/1
  Ground4/1 -> SideFrc/1
  Ground5/1 -> OverturnTrq/1
  vxtrans/1 -> Terminator1/1
  vytrans/1 -> Terminator2/1
  Rim_rotv/1 -> Terminator3/1
  InclinAngle/1 -> Terminator4/1
  muRoad/1 -> Terminator5/1
  Load/1 -> Terminator/1
  Ground1/1 -> Slp/1
  Ground6/1 -> LoadFrc/1
  Ground7/1 -> RollResist/1
  Ground8/1 -> AlignTrq/1

== system Torque_Vectoring_Schanzer20/CarMaker/IPG Vehicle/PowerTrain/Torque Vectoring System/Controller Logic1/Bicycle model ==
  steering angle : Inport
  lf : Inport  Port=2
  lr : Inport  Port=3
  velocity : Inport  Port=4
  vch^2 : Inport  Port=5
  Time delay : TransferFcn  Denominator=[0.08 1]
  linear bicycle model : Subsystem
  " desired Yaw rate" : Outport
  wires:
  lf/1 -> linear bicycle model/2(lf)
  steering angle/1 -> linear bicycle model/1(steering angle)
  lr/1 -> linear bicycle model/3(lr)
  velocity/1 -> linear bicycle model/4(velocity)
  Time delay/1 -> " desired Yaw rate"/1
  linear bicycle model/1(Yaw rate) -> Time delay/1
  vch^2/1 -> linear bicycle model/5(vch^2)

== system Torque_Vectoring_Schanzer20/CarMaker/IPG Vehicle/PowerTrain/Torque Vectoring System/Controller Logic1/Slider ==

== system Torque_Vectoring_Schanzer20/CarMaker/IPG Vehicle/PowerTrain/Torque Vectoring System/Controller Logic1/TORQUE DISTRIBUTION FRONT_REAR ==
  m : Inport
  M : Inport  Port=2
  lf : Inport  Port=3
  lr : Inport  Port=4
  lr1 : Inport  Port=5
  longitudinal acceleration : Inport  Port=6
  height center of gravity : Inport  Port=7
  Constant2 : Constant
  FRONTLOAD X : Subsystem
  LOADRATIO FRONT : Product  Inputs=*/
  LOADRATIO REAR : Sum  Inputs=+-
  REARLOAD x : Subsystem
  TOTAL WHEELLOAD : Sum
  ratioF : Outport
  ratioR : Outport  Port=2
  wires:
  REARLOAD x/1(L) -> FRONTLOAD X/5(L)
  TOTAL WHEELLOAD/1 -> LOADRATIO FRONT/2
  lf/1 -> REARLOAD x/2(lf)
  height center of gravity/1 -> REARLOAD x/5(height center of gravity), FRONTLOAD X/4(height center of gravity)
  m/1 -> FRONTLOAD X/1(m)
  FRONTLOAD X/1(normalloadF) -> TOTAL WHEELLOAD/1, LOADRATIO FRONT/1
  lr1/1 -> FRONTLOAD X/2(lr)
  M/1 -> REARLOAD x/1(M)
  lr/1 -> REARLOAD x/3(lr)
  REARLOAD x/2(normalloadR) -> TOTAL WHEELLOAD/2
  LOADRATIO FRONT/1 -> LOADRATIO REAR/2, ratioF/1
  LOADRATIO REAR/1 -> ratioR/1
  Constant2/1 -> LOADRATIO REAR/1
  longitudinal acceleration/1 -> FRONTLOAD X/3(longitudinal acceleration), REARLOAD x/4(longitudinal acceleration)

== system Torque_Vectoring_Schanzer20/CarMaker/IPG Vehicle/PowerTrain/Torque Vectoring System/Controller Logic1/Torque Vectoring ==
  desired Yaw rate : Inport
  torqueFL : Inport  Port=2
  sensor yaw rate : Inport  Port=3
  torqueRL : Inport  Port=4
  torqueFR : Inport  Port=5
  torqueRR : Inport  Port=6
  ratioF : Inport  Port=7
  ratioR : Inport  Port=8
  car.ay : Inport  Port=9
  twidth F : Inport  Port=10
  twidth R : Inport  Port=11
  Switch torque vectoring on : Subsystem
  torque distribution : Subsystem
  TORQUE LEFT FRONT : Outport
  TORQUE LEFT REAR : Outport  Port=2
  TORQUE RIGHT FRONT : Outport  Port=3
  TORQUE RIGHT REAR : Outport  Port=4
  wires:
  Switch torque vectoring on/4(RRo) -> TORQUE RIGHT REAR/1
  torque distribution/2(T,RL) -> Switch torque vectoring on/6(T,RL)
  torque distribution/4(T,RR) -> Switch torque vectoring on/8(T,RR)
  torque distribution/1(T,FL) -> Switch torque vectoring on/2(T,FL)
  Switch torque vectoring on/1(FLo) -> TORQUE LEFT FRONT/1
  desired Yaw rate/1 -> torque distribution/1("desired Yaw rate ")
  torqueFL/1 -> Switch torque vectoring on/1(tFL), torque distribution/2(torque front left)
  torque distribution/3(T,FR) -> Switch torque vectoring on/7(T,FR)
  ratioF/1 -> torque distribution/7(In9)
  torqueRR/1 -> Switch torque vectoring on/5(tRR), torque distribution/6(torque rear right)
  Switch torque vectoring on/3(FRo) -> TORQUE RIGHT FRONT/1
  Switch torque vectoring on/2(RLo) -> TORQUE LEFT REAR/1
  torqueRL/1 -> Switch torque vectoring on/3(tRL), torque distribution/4(torque rear left)
  torqueFR/1 -> Switch torque vectoring on/4(tFR), torque distribution/5(torque front right)
  sensor yaw rate/1 -> torque distribution/3(yaw rate sensor)
  ratioR/1 -> torque distribution/8(In12)
  car.ay/1 -> torque distribution/9(car.ay)
  twidth F/1 -> torque distribution/10(twidth F)
  twidth R/1 -> torque distribution/11(twidth R)

== system Torque_Vectoring_Schanzer20/CarMaker/IPG Vehicle/PowerTrain/Torque Vectoring System/activate system dependent1/If Action Subsystem ==
  In1 : Inport
  Action Port : ActionPort  ActionType=then
  Out1 : Outport
  wires:
  In1/1 -> Out1/1

== system Torque_Vectoring_Schanzer20/CarMaker/IPG Vehicle/PowerTrain/Torque Vectoring System/activate system dependent1/If Action Subsystem1 ==
  In1 : Inport
  Action Port : ActionPort  ActionType=else
  Out1 : Outport
  wires:
  In1/1 -> Out1/1

== system Torque_Vectoring_Schanzer20/CarMaker/IPG Vehicle/PowerTrain/Torque Vectoring System/activate system dependent1/If Action Subsystem2 ==
  In1 : Inport
  Action Port : ActionPort  ActionType=then
  Out1 : Outport
  wires:
  In1/1 -> Out1/1

== system Torque_Vectoring_Schanzer20/CarMaker/IPG Vehicle/PowerTrain/Torque Vectoring System/activate system dependent1/If Action Subsystem3 ==
  In1 : Inport
  Action Port : ActionPort  ActionType=else
  Out1 : Outport
  wires:
  In1/1 -> Out1/1

== system Torque_Vectoring_Schanzer20/CarMaker/IPG Vehicle/PowerTrain/Torque Vectoring System/activate system dependent2/If Action Subsystem ==
  In1 : Inport
  Action Port : ActionPort  ActionType=then
  Out1 : Outport
  wires:
  In1/1 -> Out1/1

== system Torque_Vectoring_Schanzer20/CarMaker/IPG Vehicle/PowerTrain/Torque Vectoring System/activate system dependent2/If Action Subsystem1 ==
  In1 : Inport
  Action Port : ActionPort  ActionType=else
  Out1 : Outport
  wires:
  In1/1 -> Out1/1

== system Torque_Vectoring_Schanzer20/CarMaker/IPG Vehicle/PowerTrain/Torque Vectoring System/activate system dependent2/If Action Subsystem2 ==
  In1 : Inport
  Action Port : ActionPort  ActionType=then
  Out1 : Outport
  wires:
  In1/1 -> Out1/1

== system Torque_Vectoring_Schanzer20/CarMaker/IPG Vehicle/PowerTrain/Torque Vectoring System/activate system dependent2/If Action Subsystem3 ==
  In1 : Inport
  Action Port : ActionPort  ActionType=else
  Out1 : Outport
  wires:
  In1/1 -> Out1/1

== system Torque_Vectoring_Schanzer20/CarMaker/IPG Vehicle/PowerTrain/Torque Vectoring System/activate system dependent3/If Action Subsystem ==
  In1 : Inport
  Action Port : ActionPort  ActionType=then
  Out1 : Outport
  wires:
  In1/1 -> Out1/1

== system Torque_Vectoring_Schanzer20/CarMaker/IPG Vehicle/PowerTrain/Torque Vectoring System/activate system dependent3/If Action Subsystem1 ==
  In1 : Inport
  Action Port : ActionPort  ActionType=else
  Out1 : Outport
  wires:
  In1/1 -> Out1/1

== system Torque_Vectoring_Schanzer20/CarMaker/IPG Vehicle/PowerTrain/Torque Vectoring System/activate system dependent3/If Action Subsystem2 ==
  In1 : Inport
  Action Port : ActionPort  ActionType=then
  Out1 : Outport
  wires:
  In1/1 -> Out1/1

== system Torque_Vectoring_Schanzer20/CarMaker/IPG Vehicle/PowerTrain/Torque Vectoring System/activate system dependent3/If Action Subsystem3 ==
  In1 : Inport
  Action Port : ActionPort  ActionType=else
  Out1 : Outport
  wires:
  In1/1 -> Out1/1

== system Torque_Vectoring_Schanzer20/CarMaker/IPG Vehicle/PowerTrain/Torque Vectoring System/activate system dependent5/If Action Subsystem ==
  In1 : Inport
  Action Port : ActionPort  ActionType=then
  Out1 : Outport
  wires:
  In1/1 -> Out1/1

== system Torque_Vectoring_Schanzer20/CarMaker/IPG Vehicle/PowerTrain/Torque Vectoring System/activate system dependent5/If Action Subsystem1 ==
  In1 : Inport
  Action Port : ActionPort  ActionType=else
  Out1 : Outport
  wires:
  In1/1 -> Out1/1

== system Torque_Vectoring_Schanzer20/CarMaker/IPG Vehicle/PowerTrain/Torque Vectoring System/activate system dependent5/If Action Subsystem2 ==
  In1 : Inport
  Action Port : ActionPort  ActionType=then
  Out1 : Outport
  wires:
  In1/1 -> Out1/1

== system Torque_Vectoring_Schanzer20/CarMaker/IPG Vehicle/PowerTrain/Torque Vectoring System/activate system dependent5/If Action Subsystem3 ==
  In1 : Inport
  Action Port : ActionPort  ActionType=else
  Out1 : Outport
  wires:
  In1/1 -> Out1/1

== system Torque_Vectoring_Schanzer20/CarMaker/IPG Vehicle/PowerTrain/Torque Vectoring System/activate system dependent6/If Action Subsystem ==
  In1 : Inport
  Action Port : ActionPort  ActionType=then
  Out1 : Outport
  wires:
  In1/1 -> Out1/1

== system Torque_Vectoring_Schanzer20/CarMaker/IPG Vehicle/PowerTrain/Torque Vectoring System/activate system dependent6/If Action Subsystem1 ==
  In1 : Inport
  Action Port : ActionPort  ActionType=else
  Out1 : Outport
  wires:
  In1/1 -> Out1/1

== system Torque_Vectoring_Schanzer20/CarMaker/IPG Vehicle/PowerTrain/Torque Vectoring System/activate system dependent6/If Action Subsystem2 ==
  In1 : Inport
  Action Port : ActionPort  ActionType=then
  Out1 : Outport
  wires:
  In1/1 -> Out1/1

== system Torque_Vectoring_Schanzer20/CarMaker/IPG Vehicle/PowerTrain/Torque Vectoring System/activate system dependent6/If Action Subsystem3 ==
  In1 : Inport
  Action Port : ActionPort  ActionType=else
  Out1 : Outport
  wires:
  In1/1 -> Out1/1

== system Torque_Vectoring_Schanzer20/CarMaker/IPG Vehicle/PowerTrain/Torque Vectoring System/velocity estimation/v_viaYawRate_CentrifugalAcceleration ==
  note: Assuming that angle of attack change rate is 0 -> steady state cornering (improvement would be including estimation of angle of attack (and change rate)
      | Checking of straight line noise of yaw rate sensor necessary to define a reasonable treshhold
  YawRate : Inport
  ay : Inport  Port=2
  vViaTheYawRate : Subsystem
  Out1 : Outport
  wires:
  YawRate/1 -> vViaTheYawRate/1(YawRate)
  ay/1 -> vViaTheYawRate/2(ay)
  vViaTheYawRate/1(vNew2) -> Out1/1

== system Torque_Vectoring_Schanzer20/CarMaker/IPG Vehicle/PowerTrain/Torque Vectoring System/Controller Logic1/Bicycle model/linear bicycle model ==
  note: yaw rate calculation
  steering angle : Inport
  lf : Inport  Port=2
  lr : Inport  Port=3
  velocity : Inport  Port=4
  vch^2 : Inport  Port=5
  Add : Sum
  Add1 : Sum
  Constant : Constant
  Divide1 : Product  Inputs=*/
  Divide2 : Product  Inputs=*/
  Product3 : Product
  Product4 : Product
  Scope : Scope
  Square1 : Math  Operator=square  SaturateOnIntegerOverflow=on
  Yaw rate : Outport
  wires:
  Product4/1 -> Yaw rate/1
  Product3/1 -> Divide2/2
  vch^2/1 -> Divide1/2
  Square1/1 -> Divide1/1
  Constant/1 -> Add1/1
  velocity/1 -> Divide2/1, Square1/1
  lr/1 -> Add/2
  Divide2/1 -> Product4/2
  Add1/1 -> Product3/1
  Divide1/1 -> Add1/2
  Add/1 -> Product3/2  "l"
  steering angle/1 -> Product4/1, Scope/1
  lf/1 -> Add/1

== system Torque_Vectoring_Schanzer20/CarMaker/IPG Vehicle/PowerTrain/Torque Vectoring System/Controller Logic1/TORQUE DISTRIBUTION FRONT_REAR/FRONTLOAD X ==
  m : Inport
  lr : Inport  Port=2
  longitudinal acceleration : Inport  Port=3
  height center of gravity : Inport  Port=4
  L : Inport  Port=5
  Constant4 : Constant  Value=9.81
  NORMALLOAD FRONT : Product  Inputs=*/
  Product3 : Product
  Product4 : Product
  Product5 : Product
  wheelbase3 : Sum  Inputs=-+
  normalloadF : Outport
  wires:
  Product3/1 -> wheelbase3/1
  L/1 -> NORMALLOAD FRONT/2
  Product4/1 -> wheelbase3/2
  Product5/1 -> NORMALLOAD FRONT/1
  NORMALLOAD FRONT/1 -> normalloadF/1
  Constant4/1 -> Product4/1
  wheelbase3/1 -> Product5/1
  height center of gravity/1 -> Product3/2
  longitudinal acceleration/1 -> Product3/1
  lr/1 -> Product4/2
  m/1 -> Product5/2

== system Torque_Vectoring_Schanzer20/CarMaker/IPG Vehicle/PowerTrain/Torque Vectoring System/Controller Logic1/TORQUE DISTRIBUTION FRONT_REAR/REARLOAD x ==
  M : Inport
  lf : Inport  Port=2
  lr : Inport  Port=3
  longitudinal acceleration : Inport  Port=4
  height center of gravity : Inport  Port=5
  Constant3 : Constant  Value=9.81
  NORMALLOAD REAR : Product  Inputs=*/
  Product : Product
  Product1 : Product
  Product2 : Product
  wheelbase : Sum
  wheelbase1 : Sum
  L : Outport
  normalloadR : Outport  Port=2
  wires:
  wheelbase1/1 -> Product2/1
  Constant3/1 -> Product1/1
  wheelbase/1 -> L/1, NORMALLOAD REAR/2
  Product2/1 -> NORMALLOAD REAR/1
  lr/1 -> wheelbase/2
  Product1/1 -> wheelbase1/2
  longitudinal acceleration/1 -> Product/1
  Product/1 -> wheelbase1/1
  height center of gravity/1 -> Product/2
  M/1 -> Product2/2
  NORMALLOAD REAR/1 -> normalloadR/1
  lf/1 -> wheelbase/1, Product1/2  "lf"

== system Torque_Vectoring_Schanzer20/CarMaker/IPG Vehicle/PowerTrain/Torque Vectoring System/Controller Logic1/Torque Vectoring/Switch torque vectoring on ==
  tFL : Inport
  T,FL : Inport  Port=2
  tRL : Inport  Port=3
  tFR : Inport  Port=4
  tRR : Inport  Port=5
  T,RL : Inport  Port=6
  T,FR : Inport  Port=7
  T,RR : Inport  Port=8
  Add : Sum  Inputs=+-
  Clock : Clock
  Constant : Constant  Value=4
  Switch{,1..4} (5 alike) : Switch  Criteria=u2 > Threshold  Threshold=0.5
  Switch on Torque Vectoring : Constant  Value=1.2
  Switch on Torque Vectoring1 : Constant  Value=0
  FLo : Outport
  RLo : Outport  Port=2
  FRo : Outport  Port=3
  RRo : Outport  Port=4
  wires:
  Switch2/1 -> FRo/1
  T,FL/1 -> Switch/1
  Switch4/1 -> Switch1/2, Switch2/2, Switch3/2, Switch/2
  T,RR/1 -> Switch3/1
  Switch/1 -> FLo/1
  tFL/1 -> Switch/3
  tFR/1 -> Switch2/3
  Switch1/1 -> RLo/1
  tRL/1 -> Switch1/3
  Switch3/1 -> RRo/1
  tRR/1 -> Switch3/3
  T,FR/1 -> Switch2/1
  T,RL/1 -> Switch1/1
  Clock/1 -> Add/1
  Constant/1 -> Add/2
  Add/1 -> Switch4/1
  Switch on Torque Vectoring/1 -> Switch4/2
  Switch on Torque Vectoring1/1 -> Switch4/3

== system Torque_Vectoring_Schanzer20/CarMaker/IPG Vehicle/PowerTrain/Torque Vectoring System/Controller Logic1/Torque Vectoring/torque distribution ==
  "desired Yaw rate " : Inport
  torque front left : Inport  Port=2
  yaw rate sensor : Inport  Port=3
  torque rear left : Inport  Port=4
  torque front right : Inport  Port=5
  torque rear right : Inport  Port=6
  In9 : Inport  Port=7
  In12 : Inport  Port=8
  car.ay : Inport  Port=9
  twidth F : Inport  Port=10
  twidth R : Inport  Port=11
  Feedforward_Control : Subsystem
  Front/Rear Distribution : Subsystem
  Torque Distribution : Subsystem
  feedback control : Subsystem
  T,FL : Outport
  T,RL : Outport  Port=2
  T,FR : Outport  Port=3
  T,RR : Outport  Port=4
  wires:
  In9/1 -> Front/Rear Distribution/1(In9)
  In12/1 -> Front/Rear Distribution/2(In12)
  yaw rate sensor/1 -> feedback control/2(yaw rate sensor)
  Feedforward_Control/1(Incr_Left) -> Torque Distribution/1(LEFTratio)
  Feedforward_Control/2(Incr_Right) -> Torque Distribution/2(RIGHTratio)
  feedback control/1(Tfront) -> Torque Distribution/3(TorqueF)
  feedback control/2(Trear) -> Torque Distribution/4(TorqueR)
  torque front left/1 -> Torque Distribution/5(tFL)
  torque rear left/1 -> Torque Distribution/6(tRL)
  torque front right/1 -> Torque Distribution/7(tFR)
  torque rear right/1 -> Torque Distribution/8(tRR)
  Torque Distribution/1(TFL) -> T,FL/1
  feedback control/3(yaw sensor) -> Feedforward_Control/1(yaw sensor)
  Front/Rear Distribution/1(front) -> feedback control/3(ratioF)
  Front/Rear Distribution/2(rear) -> feedback control/4(ratioR)
  Torque Distribution/2(TFR) -> T,FR/1
  Torque Distribution/3(TRL) -> T,RL/1
  Torque Distribution/4(TRR) -> T,RR/1
  "desired Yaw rate "/1 -> feedback control/1(desired Yaw rate rad/s)
  car.ay/1 -> Feedforward_Control/2(car.ay)
  twidth F/1 -> feedback control/5(twidth F)
  twidth R/1 -> feedback control/6(twidth R)

== system Torque_Vectoring_Schanzer20/CarMaker/IPG Vehicle/PowerTrain/Torque Vectoring System/velocity estimation/v_viaYawRate_CentrifugalAcceleration/vViaTheYawRate ==
  YawRate : Inport
  ay : Inport  Port=2
  Divide : Product  Inputs=*/
  Scope2 : Scope  NumInputPorts=2
  Scope3 : Scope
  vNew2 : Outport
  wires:
  Divide/1 -> vNew2/1, Scope3/1  "v_via_yaw"
  YawRate/1 -> Scope2/1, Divide/2  "YawRate"
  ay/1 -> Divide/1, Scope2/2  "ay"

== system Torque_Vectoring_Schanzer20/CarMaker/IPG Vehicle/PowerTrain/Torque Vectoring System/Controller Logic1/Torque Vectoring/torque distribution/Feedforward_Control ==
  yaw sensor : Inport
  car.ay : Inport  Port=2
  Abs : Abs
  Add : Sum
  Add7 : Sum
  Constant : Constant
  Constant7 : Constant
  Constant8 : Constant
  Divide : Product  Inputs=*/
  Gain1 : Gain  Gain=-1
  Switch : Switch  Criteria=u2 > Threshold  Threshold=0.00001
  limit torque distribution : Saturate  UpperLimit=0.7  LowerLimit=-0.7
  limit torque distribution1 : Saturate  UpperLimit=0.7  LowerLimit=-0.7
  Incr_Left : Outport
  Incr_Right : Outport  Port=2
  wires:
  Constant7/1 -> Add/2
  Constant8/1 -> Add7/2
  Add/1 -> Incr_Right/1
  Gain1/1 -> Add7/1
  limit torque distribution1/1 -> Gain1/1
  Add7/1 -> Incr_Left/1
  Switch/1 -> limit torque distribution1/1, limit torque distribution/1
  yaw sensor/1 -> Abs/1
  Abs/1 -> Switch/2
  limit torque distribution/1 -> Add/1
  Constant/1 -> Divide/2
  Divide/1 -> Switch/1
  car.ay/1 -> Divide/1

== system Torque_Vectoring_Schanzer20/CarMaker/IPG Vehicle/PowerTrain/Torque Vectoring System/Controller Logic1/Torque Vectoring/torque distribution/Front//Rear Distribution ==
  In9 : Inport
  In12 : Inport  Port=2
  Add1 : Sum
  Add5 : Sum
  Constant : Constant  Value=0.52
  Constant1 : Constant  Value=0.48
  front : Outport
  rear : Outport  Port=2
  wires:
  Add5/1 -> rear/1
  In12/1 -> Add5/1
  Constant1/1 -> Add5/2
  In9/1 -> Add1/1
  Add1/1 -> front/1
  Constant/1 -> Add1/2

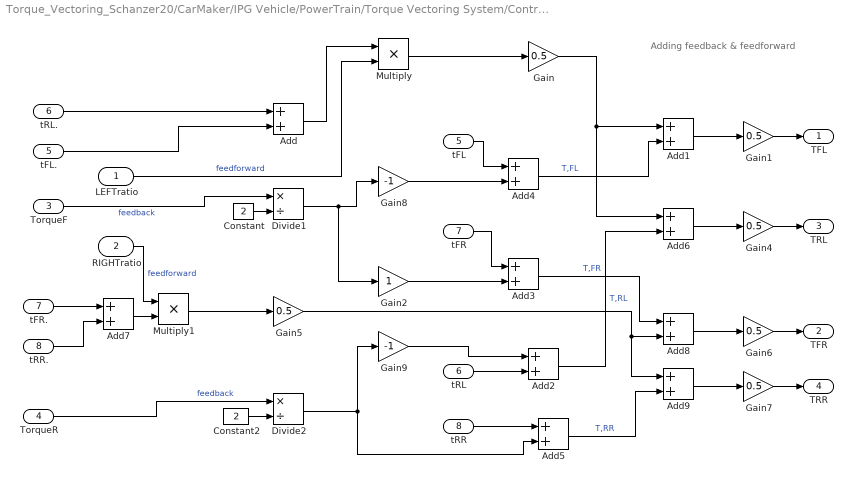
== system Torque_Vectoring_Schanzer20/CarMaker/IPG Vehicle/PowerTrain/Torque Vectoring System/Controller Logic1/Torque Vectoring/torque distribution/Torque Distribution ==
  note: Adding feedback & feedforward
  LEFTratio : Inport
  RIGHTratio : Inport  Port=2
  TorqueF : Inport  Port=3
  TorqueR : Inport  Port=4
  tFL : Inport  Port=5
  tRL : Inport  Port=6
  tFR : Inport  Port=7
  tRR : Inport  Port=8
  Add{,1..9} (10 alike) : Sum
  Constant : Constant  Value=2
  Constant2 : Constant  Value=2
  Divide1 : Product  Inputs=*/
  Divide2 : Product  Inputs=*/
  Gain{,1,4..7} (6 alike) : Gain  Gain=0.5
  Gain2 : Gain
  Gain8 : Gain  Gain=-1
  Gain9 : Gain  Gain=-1
  Multiply : Product
  Multiply1 : Product
  tFL. : InportShadow  Port=5
  tFR. : InportShadow  Port=7
  tRL. : InportShadow  Port=6
  tRR. : InportShadow  Port=8
  TFL : Outport
  TFR : Outport  Port=2
  TRL : Outport  Port=3
  TRR : Outport  Port=4
  wires:
  Add5/1 -> Add9/2  "T,RR"
  Add2/1 -> Add6/2  "T,RL"
  Add3/1 -> Add8/1  "T,FR"
  Add4/1 -> Add1/2  "T,FL"
  tRR/1 -> Add5/1
  tFL/1 -> Add4/1
  TorqueF/1 -> Divide1/1  "feedback"
  Constant2/1 -> Divide2/2
  TorqueR/1 -> Divide2/1  "feedback"
  RIGHTratio/1 -> Multiply1/1  "feedforward"
  LEFTratio/1 -> Multiply/2  "feedforward"
  tFR/1 -> Add3/1
  tRL/1 -> Add2/2
  Constant/1 -> Divide1/2
  Divide1/1 -> Gain8/1, Gain2/1
  Gain2/1 -> Add3/2
  Divide2/1 -> Add5/2, Gain9/1
  tFL./1 -> Add/2
  tRL./1 -> Add/1
  Add/1 -> Multiply/1
  Multiply/1 -> Gain/1
  Gain/1 -> Add6/1, Add1/1
  Add1/1 -> Gain1/1
  Gain1/1 -> TFL/1
  Add6/1 -> Gain4/1
  Gain4/1 -> TRL/1
  tFR./1 -> Add7/1
  tRR./1 -> Add7/2
  Add7/1 -> Multiply1/2
  Multiply1/1 -> Gain5/1
  Gain5/1 -> Add9/1, Add8/2
  Add8/1 -> Gain6/1
  Gain6/1 -> TFR/1
  Add9/1 -> Gain7/1
  Gain7/1 -> TRR/1
  Gain8/1 -> Add4/2
  Gain9/1 -> Add2/1
